simulink model "assignment_test_tmp"  (Simulink 8.3)
settings: Solver=ode45  StartTime=0.0  StopTime=10.0  RelTol=1e-3
settings Model: Creator=arnaud  LastModifiedBy=hbourbou
settings DataIOCC: SaveFormat=Structure  SignalLoggingSaveFormat=Dataset
settings DebuggingCC: UnderspecifiedInitializationDetection=Simplified  MergeDetectMultiDrivingBlocksExec=error  FrameProcessingCompatibilityMsg=error  StateNameClashWarn=none
settings GRTTargetCC: CombineOutputUpdateFcns=on  GRTInterface=off

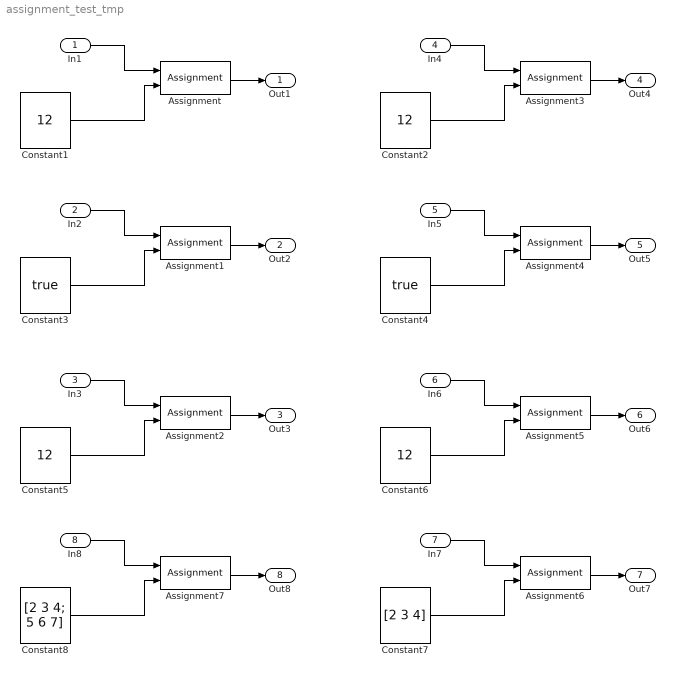
== system assignment_test_tmp ==
  In1 : Inport  PortDimensions=[2 3]
  In2 : Inport  Port=2  OutDataTypeStr=boolean  PortDimensions=[2 3]
  In3 : Inport  Port=3  OutDataTypeStr=int16  PortDimensions=[2 3]
  In4 : Inport  Port=4  PortDimensions=3
  In5 : Inport  Port=5  OutDataTypeStr=boolean  PortDimensions=3
  In6 : Inport  Port=6  OutDataTypeStr=int16  PortDimensions=3
  In7 : Inport  Port=7  OutDataTypeStr=int16  PortDimensions=3
  In8 : Inport  Port=8  OutDataTypeStr=int16  PortDimensions=[2 3]
  Assignment : Assignment  NumberOfDimensions=2  DiagnosticForDimensions=Warning  IndexOptions=Index vector (dialog),Index vector (dialog)  Indices=[1 2],2  OutputSizes=1,1
  Assignment1 : Assignment  NumberOfDimensions=2  DiagnosticForDimensions=Warning  IndexOptions=Index vector (dialog),Index vector (dialog)  Indices=[2 1],2  OutputSizes=1,1
  Assignment2 : Assignment  NumberOfDimensions=2  IndexMode=Zero-based  DiagnosticForDimensions=Warning  IndexOptions=Assign all,Index vector (dialog)  Indices=1,1  OutputSizes=1,1
  Assignment3 : Assignment  DiagnosticForDimensions=Warning  IndexOptions=Index vector (dialog)  Indices=[2 1]  OutputSizes=1
  Assignment4 : Assignment  IndexMode=Zero-based  DiagnosticForDimensions=Warning  IndexOptions=Index vector (dialog)  Indices=2  OutputSizes=1
  Assignment5 : Assignment  DiagnosticForDimensions=Warning  IndexOptions=Index vector (dialog)  Indices=1  OutputSizes=1
  Assignment6 : Assignment  DiagnosticForDimensions=Warning  IndexOptions=Assign all  Indices=1  OutputSizes=1
  Assignment7 : Assignment  NumberOfDimensions=2  DiagnosticForDimensions=Warning  IndexOptions=Assign all,Assign all  Indices=1,2  OutputSizes=1,1
  Constant1 : Constant  Value=12
  Constant2 : Constant  Value=12
  Constant3 : Constant  Value=true
  Constant4 : Constant  Value=true
  Constant5 : Constant  Value=12  OutDataTypeStr=int16
  Constant6 : Constant  Value=12  OutDataTypeStr=int16
  Constant7 : Constant  Value=[2 3 4]  OutDataTypeStr=int16
  Constant8 : Constant  Value=[2 3 4; 5 6 7]  OutDataTypeStr=int16
  Out1 : Outport
  Out2 : Outport  Port=2
  Out3 : Outport  Port=3
  Out4 : Outport  Port=4
  Out5 : Outport  Port=5
  Out6 : Outport  Port=6
  Out7 : Outport  Port=7
  Out8 : Outport  Port=8
  wires:
  Assignment/1 -> Out1/1
  In1/1 -> Assignment/1
  Constant1/1 -> Assignment/2
  Assignment1/1 -> Out2/1
  In2/1 -> Assignment1/1
  Constant3/1 -> Assignment1/2
  Assignment2/1 -> Out3/1
  In3/1 -> Assignment2/1
  Constant5/1 -> Assignment2/2
  Assignment3/1 -> Out4/1
  In4/1 -> Assignment3/1
  Constant2/1 -> Assignment3/2
  Assignment4/1 -> Out5/1
  In5/1 -> Assignment4/1
  Constant4/1 -> Assignment4/2
  Assignment5/1 -> Out6/1
  In6/1 -> Assignment5/1
  Constant6/1 -> Assignment5/2
  Assignment6/1 -> Out7/1
  In7/1 -> Assignment6/1
  Constant7/1 -> Assignment6/2
  Assignment7/1 -> Out8/1
  In8/1 -> Assignment7/1
  Constant8/1 -> Assignment7/2
